simulink model "PlantModel_"  (R2018b)
settings: Solver=VariableStepAuto  StartTime=0.0  StopTime=10.0  RelTol=1e-3
values from neighbouring files (symbols this model uses):
  A = [0 0 0 0 1 0 0 0 0 0 0 0 ... (64 elements, 8x8)]    [IC_4DOF_new.mat]
  a1_dim = 0.409090909091    [IC_4DOF_new.mat]
  a2_dim = 0.409090909091    [IC_4DOF_new.mat]
  alpha1 = 0    [IC_4DOF_new.mat]
  Ax_dim = 0.000833333333333    [IC_4DOF_new.mat]
  beta1 = 0    [IC_4DOF_new.mat]
  C_ss = [1 0 0 0 0 1 0 0 0 0 1 0 ... (32 elements, 4x8)]    [IC_4DOF_new.mat]
  D_ss = [0 0 0 0 0 0 0 0 0 0 0 0 ... (16 elements, 4x4)]    [IC_4DOF_new.mat]
  delta_dim = 1    [IC_4DOF_new.mat]
  omega_dim = 0.753327454075    [IC_4DOF_new.mat]
  P2 = 8.714    [IC_4DOF_new.mat]
  p_dim = 0    [IC_4DOF_new.mat]
  Pk = 1000000    [IC_4DOF_new.mat]
  Px_dim = 0    [IC_4DOF_new.mat]
  x1 = 0.5    [IC_4DOF_new.mat]
  y1 = 0.25    [IC_4DOF_new.mat]
  zer_o = [0 0 0 0]    [IC_4DOF_new.mat]
libraries: dspmtrx3 x2, cstblocks x1
settings Model: Creator=first  LastModifiedBy=first
settings DebuggingCC: UnderSpecifiedDimensionMsg=warning

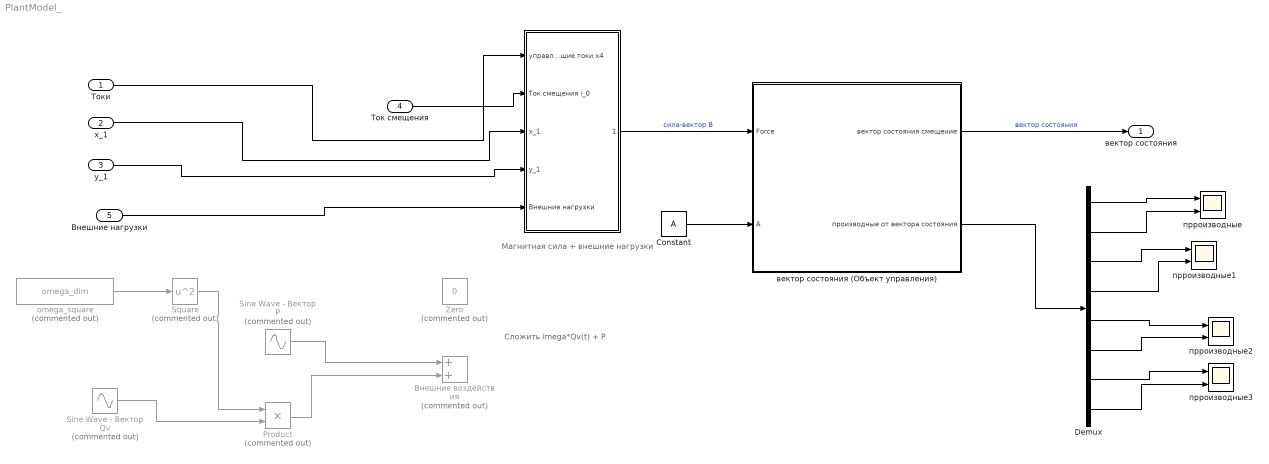
== system PlantModel_ ==
  note: Магнитная сила + внешние нагрузки
  note: Сложить imega*Qv(t) + P
  Токи : Inport
  x_1 : Inport  Port=2
  y_1 : Inport  Port=3
  Ток смещения : Inport  Port=4
  Внешние нагрузки : Inport  Port=5
  " " : Subsystem
  " вектор состояния (Объект управления) " : Subsystem
  Constant : Constant  Value=A
  Demux : Demux  Outputs=8
  Product : Product  Commented=on
  Sine Wave - Вектор P : Sin  Commented=on  Amplitude=Ax_dim  Bias=Px_dim  Frequency=p_dim  SampleTime=1
  Sine Wave - Вектор Qv : Sin  Commented=on  Amplitude=Ax_dim  Bias=Px_dim  Frequency=p_dim  SampleTime=1
  Square : Math  Commented=on  Operator=square  SaturateOnIntegerOverflow=on
  Zero : Constant  Commented=on  Value=0  OutDataTypeStr=Inherit: Inherit via back propagation
  omega_square : Constant  Commented=on  Value=omega_dim
  Внешние воздействия : Sum  Commented=on
  прроизводные{,1..3} (4 alike) : Scope  NumInputPorts=2
  вектор состояния : Outport
  wires:
  omega_square/1 -> Square/1
  Constant/1 -> " вектор состояния (Объект управления) "/2("A ")
  Square/1 -> Product/1
  Product/1 -> Внешние воздействия/2
  Токи/1 -> " "/1(управляющие токи x4)
  " вектор состояния (Объект управления) "/1(вектор состояния смещение) -> вектор состояния/1  "вектор состояния"
  " "/1(" ") -> " вектор состояния (Объект управления) "/1(Force)  "сила-вектор B"
  Sine Wave - Вектор Qv/1 -> Product/2
  Sine Wave - Вектор P/1 -> Внешние воздействия/1
  x_1/1 -> " "/3(x_1)
  y_1/1 -> " "/4(y_1)
  Ток смещения/1 -> " "/2(Ток смещения i_0)
  " вектор состояния (Объект управления) "/2(производные от вектора состояния) -> Demux/1
  Demux/2 -> прроизводные/2
  Demux/1 -> прроизводные/1
  Demux/3 -> прроизводные1/1
  Demux/4 -> прроизводные1/2
  Demux/5 -> прроизводные2/1
  Demux/6 -> прроизводные2/2
  Demux/7 -> прроизводные3/1
  Demux/8 -> прроизводные3/2
  Внешние нагрузки/1 -> " "/5(Внешние нагрузки)

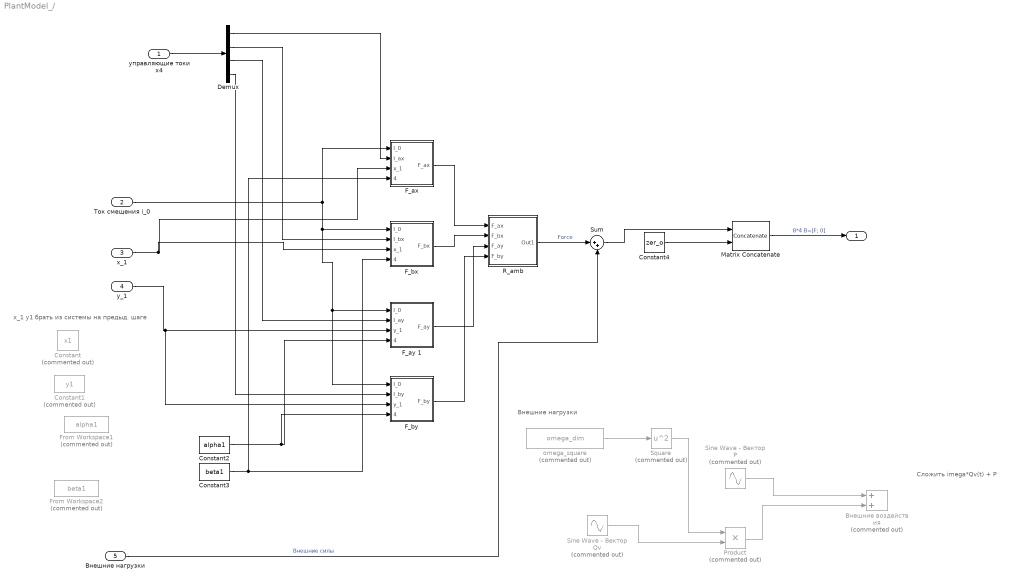
== system PlantModel_/  ==
  note: Внешние нагрузки
  note: x_1 y1 брать из системы на предыд. шаге
  note: Сложить imega*Qv(t) + P
  управляющие токи x4 : Inport
  Ток смещения i_0 : Inport  Port=2
  x_1 : Inport  Port=3
  y_1 : Inport  Port=4
  Внешние нагрузки : Inport  Port=5
  Constant : Constant  Commented=on  Value=x1
  Constant1 : Constant  Commented=on  Value=y1
  Constant2 : Constant  Value=alpha1
  Constant3 : Constant  Value=beta1
  Constant4 : Constant  Value=zer_o
  Demux : Demux
  F_ax : Subsystem
  F_ay 1 : Subsystem
  F_bx : Subsystem
  F_by : Subsystem
  From Workspace1 : FromWorkspace  Commented=on  VariableName=alpha1  SampleTime=0
  From Workspace2 : FromWorkspace  Commented=on  VariableName=beta1  SampleTime=0
  Matrix Concatenate : Concatenate  Mode=Multidimensional array
  Product : Product  Commented=on
  R_amb : Subsystem
  Sine Wave - Вектор P : Sin  Commented=on  Amplitude=Ax_dim  Bias=Px_dim  Frequency=p_dim  SampleTime=1
  Sine Wave - Вектор Qv : Sin  Commented=on  Amplitude=Ax_dim  Bias=Px_dim  Frequency=p_dim  SampleTime=1
  Square : Math  Commented=on  Operator=square  SaturateOnIntegerOverflow=on
  Sum : Sum  Inputs=|++
  omega_square : Constant  Commented=on  Value=omega_dim
  Внешние воздействия : Sum  Commented=on
  " " : Outport
  wires:
  F_ax/1(F_ax) -> R_amb/1(F_ax)
  F_bx/1(F_bx) -> R_amb/2(F_bx)
  F_ay 1/1(F_ay) -> R_amb/3(F_ay)
  F_by/1(F_by) -> R_amb/4(F_by)
  Ток смещения i_0/1 -> F_by/1(I_0), F_ay 1/1(I_0), F_bx/1(I_0), F_ax/1(I_0)
  управляющие токи x4/1 -> Demux/1
  Demux/1 -> F_ax/2(I_ax)
  Demux/2 -> F_bx/2(I_bx)
  Demux/3 -> F_ay 1/2(I_ay)
  Demux/4 -> F_by/2(I_by)
  Constant2/1 -> F_by/4(alpha_1), F_ay 1/4(alpha_1)
  Constant3/1 -> F_bx/4(betta_1), F_ax/4(betta_1)
  Matrix Concatenate/1 -> " "/1  "8*4 B=[F; 0]"
  Constant4/1 -> Matrix Concatenate/2
  x_1/1 -> F_bx/3(x_1), F_ax/3(x_1)
  y_1/1 -> F_by/3(y_1), F_ay 1/3(y_1)
  R_amb/1(Out1) -> Sum/1  "Force"
  omega_square/1 -> Square/1
  Sine Wave - Вектор P/1 -> Внешние воздействия/1
  Square/1 -> Product/1
  Sine Wave - Вектор Qv/1 -> Product/2
  Product/1 -> Внешние воздействия/2
  Sum/1 -> Matrix Concatenate/1
  Внешние нагрузки/1 -> Sum/2  "Внешние силы"

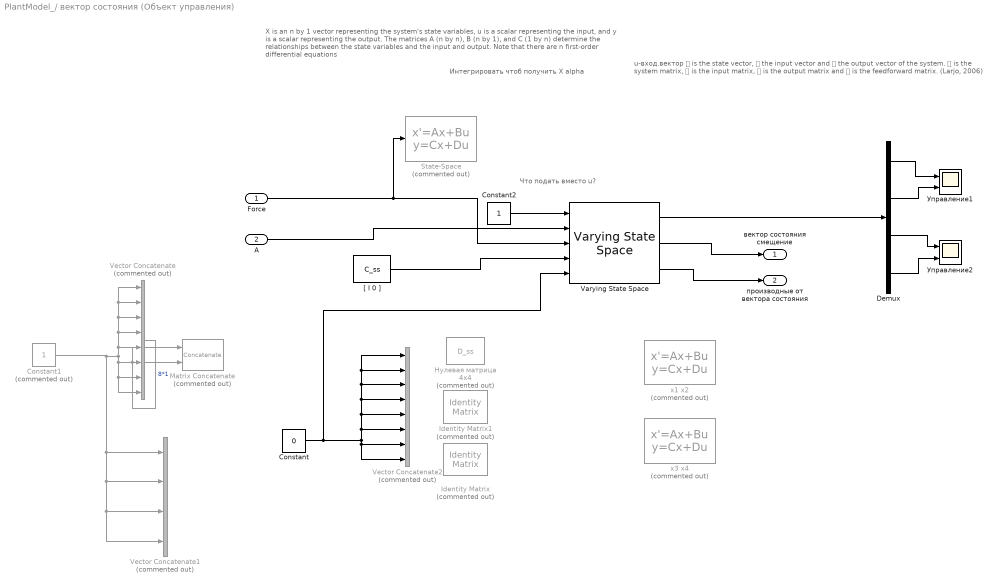
== system PlantModel_/ вектор состояния (Объект управления)  ==
  note: Что подать вместо u?
  note: u-вход.вектор
      |  𝒙 is the state vector, 𝒖 the input vector and 𝒚 the output vector of the system.
      | 𝐀 is the system matrix, 𝐁 is the input matrix, 𝐂 is the output matrix and 𝐃 is the feedforward matrix.
      | (Larjo, 2006)
  note: X is an n by 1 vector representing the system's state variables, u is a scalar representing the input, and y is a scalar representing the output.
      |  The matrices A (n by n), B (n by 1), and C (1 by n) determine the relationships between the state variables and the input and output.
      | Note that there are n first-order differential equations
  note: Интегрировать чтоб получить X alpha
  Force : Inport
  "A " : Inport  Port=2
  Constant : Constant  Value=0
  Constant1 : Constant  Commented=on
  Constant2 : Constant
  Demux : Demux
  Identity Matrix : dspmtrx3/Identity Matrix  Commented=on  Inherit=off  N=4  Ts=1  dataType=double  isSigned=on  wordLen=16  udDataType=sfix(16)  fracBitsMode=Best precision  numFracBits=15  OutDataTypeStr=double  LastOutDataTypeStr=double
      settings: SourceProductName=DSP System Toolbox
  Identity Matrix1 : dspmtrx3/Identity Matrix  Commented=on  Inherit=off  N=8  Ts=1  dataType=double  isSigned=on  wordLen=16  udDataType=sfix(16)  fracBitsMode=Best precision  numFracBits=15  OutDataTypeStr=double  LastOutDataTypeStr=double
      settings: SourceProductName=DSP System Toolbox
  Matrix Concatenate : Concatenate  Commented=on  Mode=Multidimensional array  ConcatenateDimension=8
  State-Space : StateSpace  Commented=on  InitialCondition=0
  Varying State Space : cstblocks/Linear Parameter Varying/Varying State Space  x0=0  xNames=''  OutputX=on  OutputDX=on
      settings: SourceProductName=Control System Toolbox
  Vector Concatenate : Concatenate  Commented=on  NumInputs=8
  Vector Concatenate1 : Concatenate  Commented=on  NumInputs=4
  Vector Concatenate2 : Concatenate  Commented=on  NumInputs=8
  "[ I 0 ] " : Constant  Value=C_ss
  x1 x2 : StateSpace  Commented=on  InitialCondition=0
  x3 x4 : StateSpace  Commented=on  InitialCondition=0
  Нулевая матрица 4x4 : Constant  Commented=on  Value=D_ss
  Управление1 : Scope  NumInputPorts=2
  Управление2 : Scope  NumInputPorts=2
  вектор состояния смещение : Outport
  производные от вектора состояния : Outport  Port=2
  wires:
  Force/1 -> Varying State Space/3, State-Space/1
  "A "/1 -> Varying State Space/2
  Varying State Space/3 -> производные от вектора состояния/1
  Constant1/1 -> Vector Concatenate1/4, Vector Concatenate1/3, Vector Concatenate1/2, Vector Concatenate1/1, Vector Concatenate/4, Vector Concatenate/1, Vector Concatenate/2, Vector Concatenate/3, Vector Concatenate/5, Vector Concatenate/8, Vector Concatenate/7, Vector Concatenate/6
  Vector Concatenate/1 -> Matrix Concatenate/1, Matrix Concatenate/2  "8*1"
  Constant/1 -> Varying State Space/5, Vector Concatenate2/8, Vector Concatenate2/7, Vector Concatenate2/6, Vector Concatenate2/4, Vector Concatenate2/3, Vector Concatenate2/2, Vector Concatenate2/1, Vector Concatenate2/5
  Varying State Space/2 -> вектор состояния смещение/1
  "[ I 0 ] "/1 -> Varying State Space/4
  Constant2/1 -> Varying State Space/1
  Demux/3 -> Управление2/1
  Varying State Space/1 -> Demux/1
  Demux/1 -> Управление1/1
  Demux/2 -> Управление1/2
  Demux/4 -> Управление2/2

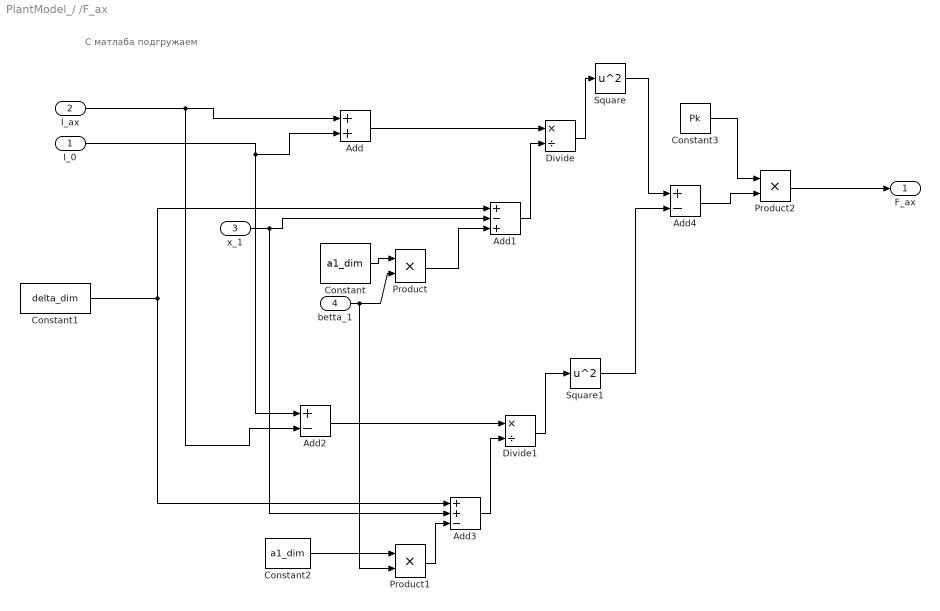
== system PlantModel_/ /F_ax ==
  note: С матлаба подгружаем
  I_0 : Inport
  I_ax : Inport  Port=2
  x_1 : Inport  Port=3
  betta_1 : Inport  Port=4
  Add : Sum
  Add1 : Sum  Inputs=+-+
  Add2 : Sum  Inputs=+-
  Add3 : Sum  Inputs=++-
  Add4 : Sum  Inputs=+-
  Constant : Constant  Value=a1_dim
  Constant1 : Constant  Value=delta_dim
  Constant2 : Constant  Value=a1_dim
  Constant3 : Constant  Value=Pk
  Divide : Product  Inputs=*/
  Divide1 : Product  Inputs=*/
  Product : Product
  Product1 : Product
  Product2 : Product
  Square : Math  Operator=square  SaturateOnIntegerOverflow=on
  Square1 : Math  Operator=square  SaturateOnIntegerOverflow=on
  F_ax : Outport
  wires:
  Product2/1 -> F_ax/1
  Constant/1 -> Product/1
  Product/1 -> Add1/3
  Add1/1 -> Divide/2
  Add/1 -> Divide/1
  Divide/1 -> Square/1
  Product1/1 -> Add3/3
  Add2/1 -> Divide1/1
  Constant2/1 -> Product1/1
  I_ax/1 -> Add2/2, Add/1
  Add3/1 -> Divide1/2
  x_1/1 -> Add1/2, Add3/2
  Divide1/1 -> Square1/1
  I_0/1 -> Add/2, Add2/1
  betta_1/1 -> Product/2, Product1/2
  Square/1 -> Add4/1
  Square1/1 -> Add4/2
  Constant3/1 -> Product2/1
  Add4/1 -> Product2/2
  Constant1/1 -> Add1/1, Add3/1

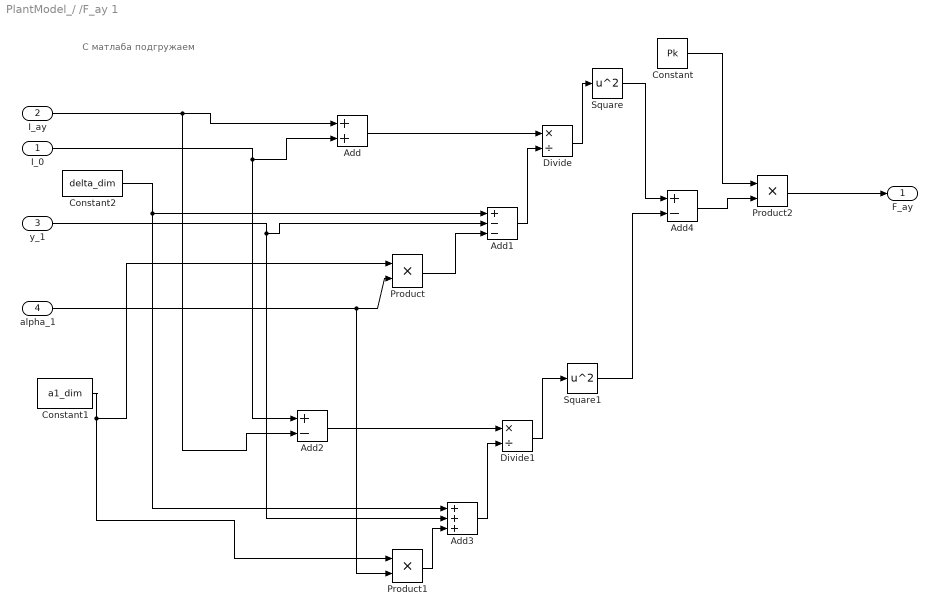
== system PlantModel_/ /F_ay 1 ==
  note: С матлаба подгружаем
  I_0 : Inport
  I_ay : Inport  Port=2
  y_1 : Inport  Port=3
  alpha_1 : Inport  Port=4
  Add : Sum
  Add1 : Sum  Inputs=+--
  Add2 : Sum  Inputs=+-
  Add3 : Sum  Inputs=+++
  Add4 : Sum  Inputs=+-
  Constant : Constant  Value=Pk
  Constant1 : Constant  Value=a1_dim
  Constant2 : Constant  Value=delta_dim
  Divide : Product  Inputs=*/
  Divide1 : Product  Inputs=*/
  Product : Product
  Product1 : Product
  Product2 : Product
  Square : Math  Operator=square  SaturateOnIntegerOverflow=on
  Square1 : Math  Operator=square  SaturateOnIntegerOverflow=on
  F_ay : Outport
  wires:
  Product2/1 -> F_ay/1
  Product/1 -> Add1/3
  Add1/1 -> Divide/2
  Add/1 -> Divide/1
  Divide/1 -> Square/1
  Product1/1 -> Add3/3
  Add2/1 -> Divide1/1
  Constant1/1 -> Product1/1, Product/1
  I_ay/1 -> Add2/2, Add/1
  Add3/1 -> Divide1/2
  y_1/1 -> Add1/2, Add3/2
  Divide1/1 -> Square1/1
  I_0/1 -> Add/2, Add2/1
  alpha_1/1 -> Product/2, Product1/2
  Square/1 -> Add4/1
  Square1/1 -> Add4/2
  Constant/1 -> Product2/1
  Add4/1 -> Product2/2
  Constant2/1 -> Add3/1, Add1/1

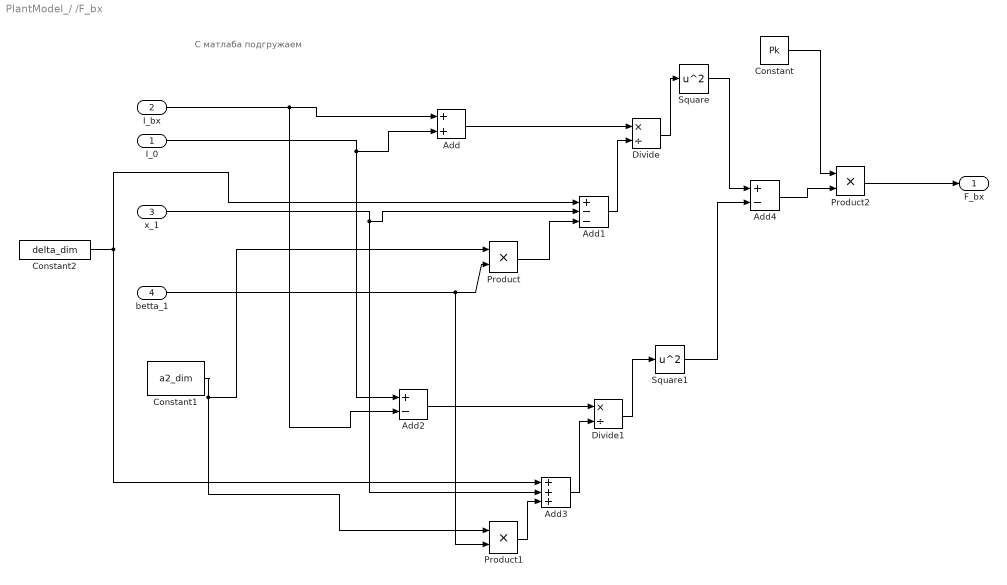
== system PlantModel_/ /F_bx ==
  note: С матлаба подгружаем
  I_0 : Inport
  I_bx : Inport  Port=2
  x_1 : Inport  Port=3
  betta_1 : Inport  Port=4
  Add : Sum
  Add1 : Sum  Inputs=+--
  Add2 : Sum  Inputs=+-
  Add3 : Sum  Inputs=+++
  Add4 : Sum  Inputs=+-
  Constant : Constant  Value=Pk
  Constant1 : Constant  Value=a2_dim
  Constant2 : Constant  Value=delta_dim
  Divide : Product  Inputs=*/
  Divide1 : Product  Inputs=*/
  Product : Product
  Product1 : Product
  Product2 : Product
  Square : Math  Operator=square  SaturateOnIntegerOverflow=on
  Square1 : Math  Operator=square  SaturateOnIntegerOverflow=on
  F_bx : Outport
  wires:
  Product2/1 -> F_bx/1
  Product/1 -> Add1/3
  Add1/1 -> Divide/2
  Add/1 -> Divide/1
  Divide/1 -> Square/1
  Product1/1 -> Add3/3
  Add2/1 -> Divide1/1
  Constant1/1 -> Product1/1, Product/1
  I_bx/1 -> Add2/2, Add/1
  Add3/1 -> Divide1/2
  x_1/1 -> Add1/2, Add3/2
  Divide1/1 -> Square1/1
  I_0/1 -> Add/2, Add2/1
  betta_1/1 -> Product/2, Product1/2
  Square/1 -> Add4/1
  Square1/1 -> Add4/2
  Constant/1 -> Product2/1
  Add4/1 -> Product2/2
  Constant2/1 -> Add1/1, Add3/1

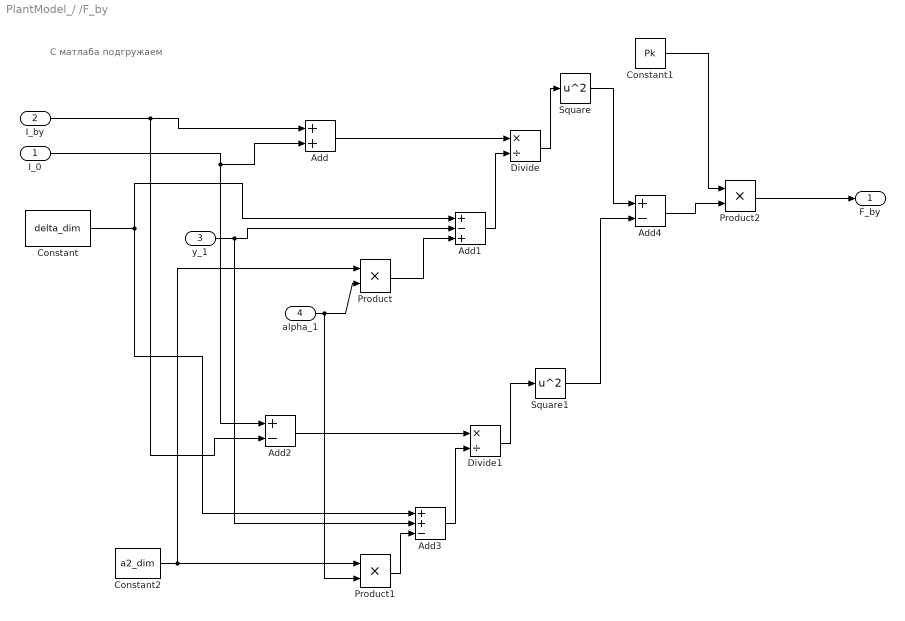
== system PlantModel_/ /F_by ==
  note: С матлаба подгружаем
  I_0 : Inport
  I_by : Inport  Port=2
  y_1 : Inport  Port=3
  alpha_1 : Inport  Port=4
  Add : Sum
  Add1 : Sum  Inputs=+-+
  Add2 : Sum  Inputs=+-
  Add3 : Sum  Inputs=++-
  Add4 : Sum  Inputs=+-
  Constant : Constant  Value=delta_dim
  Constant1 : Constant  Value=Pk
  Constant2 : Constant  Value=a2_dim
  Divide : Product  Inputs=*/
  Divide1 : Product  Inputs=*/
  Product : Product
  Product1 : Product
  Product2 : Product
  Square : Math  Operator=square  SaturateOnIntegerOverflow=on
  Square1 : Math  Operator=square  SaturateOnIntegerOverflow=on
  F_by : Outport
  wires:
  Product2/1 -> F_by/1
  Constant2/1 -> Product/1, Product1/1
  Product/1 -> Add1/3
  Add1/1 -> Divide/2
  Add/1 -> Divide/1
  Divide/1 -> Square/1
  Product1/1 -> Add3/3
  Add2/1 -> Divide1/1
  I_by/1 -> Add2/2, Add/1
  Add3/1 -> Divide1/2
  y_1/1 -> Add1/2, Add3/2
  Constant/1 -> Add1/1, Add3/1
  Divide1/1 -> Square1/1
  I_0/1 -> Add/2, Add2/1
  alpha_1/1 -> Product/2, Product1/2
  Square/1 -> Add4/1
  Square1/1 -> Add4/2
  Constant1/1 -> Product2/1
  Add4/1 -> Product2/2

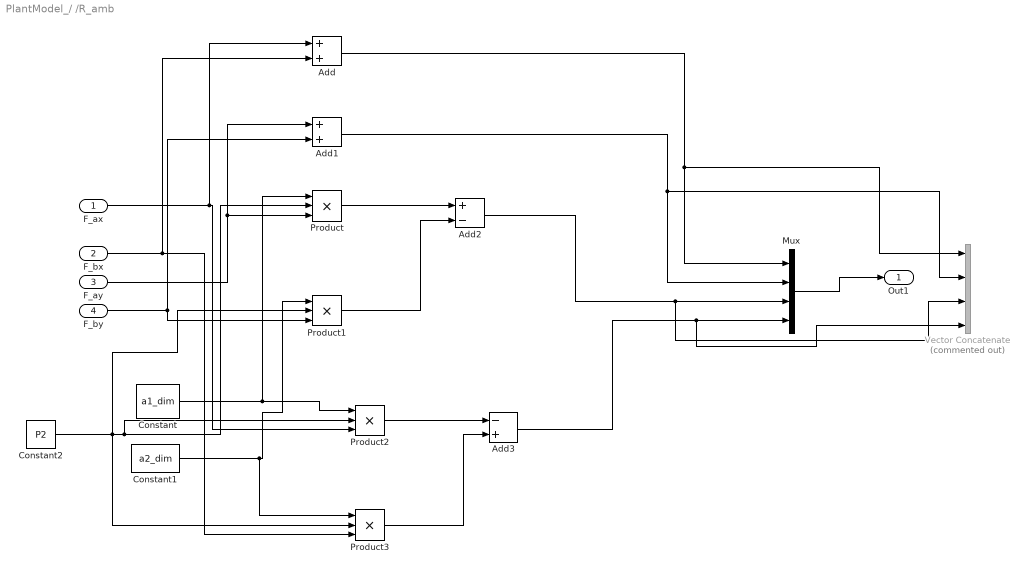
== system PlantModel_/ /R_amb ==
  F_ax : Inport
  F_bx : Inport  Port=2
  F_ay : Inport  Port=3
  F_by : Inport  Port=4
  Add : Sum
  Add1 : Sum
  Add2 : Sum  Inputs=+-
  Add3 : Sum  Inputs=-+
  Constant : Constant  Value=a1_dim
  Constant1 : Constant  Value=a2_dim
  Constant2 : Constant  Value=P2
  Mux : Mux
  Product{,1..3} (4 alike) : Product  Inputs=3
  Vector Concatenate : Concatenate  Commented=on  NumInputs=4
  Out1 : Outport  PortDimensions=4
  wires:
  F_ax/1 -> Product2/3, Add/1
  F_bx/1 -> Product3/3, Add/2
  Add/1 -> Mux/1, Vector Concatenate/1
  F_ay/1 -> Product/3, Add1/1
  F_by/1 -> Product1/3, Add1/2
  Add1/1 -> Mux/2, Vector Concatenate/2
  Constant/1 -> Product2/1, Product/1
  Product/1 -> Add2/1
  Constant1/1 -> Product3/1, Product1/1
  Product1/1 -> Add2/2
  Add2/1 -> Vector Concatenate/3, Mux/3
  Product3/1 -> Add3/2
  Product2/1 -> Add3/1
  Add3/1 -> Vector Concatenate/4, Mux/4
  Constant2/1 -> Product/2, Product2/2, Product3/2, Product1/2
  Mux/1 -> Out1/1
